simulink model "gm_sampleModel1743_4_sub"  (R2023a)
settings: Solver=VariableStepAuto  StartTime=0.0  StopTime=10.0  RelTol=1e-3
libraries: hdlsllib x3, simulink x2
settings Model: Creator=user1  LastModifiedBy=user1
settings OptimizationCC: BlockReduction=off  ConditionallyExecuteInputs=off
settings DebuggingCC: InheritedTsInSrcMsg=none

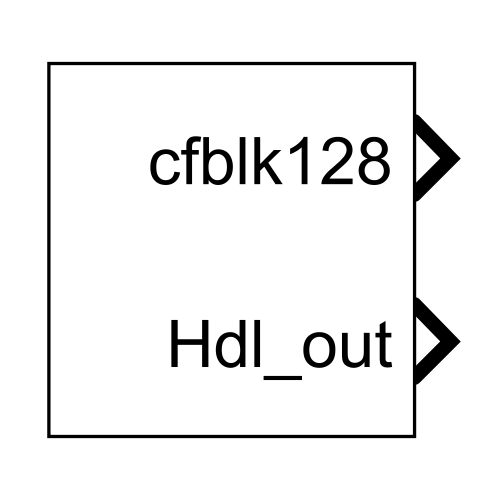
[thumbnail: Simulink's stored preview of the top-level diagram]
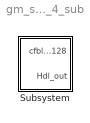
== system gm_sampleModel1743_4_sub ==
  Subsystem : Subsystem

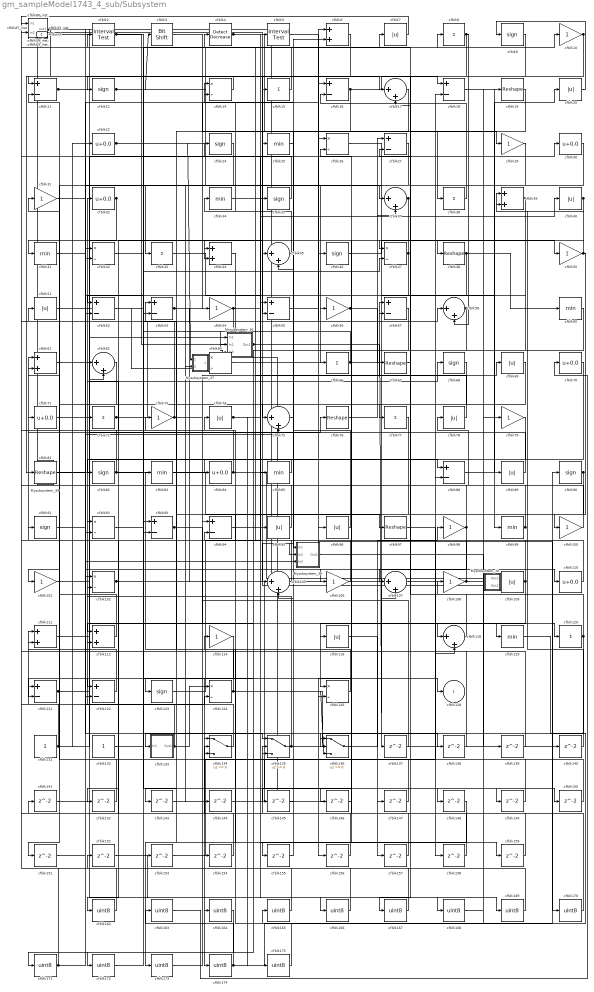
== system gm_sampleModel1743_4_sub/Subsystem ==
  Mysubsystem_16 : Subsystem
  Mysubsystem_19 : Subsystem
  Mysubsystem_36 : Subsystem
  Mysubsystem_37 : Subsystem
  Mysubsystem_39 : Subsystem
  cfblk{10,29,31,50,54,56,73,79,98,100..101,106,108,114} (14 alike) : Gain  OutDataTypeStr=uint8
  cfblk{14,26,42,47,64,92,102,124,126} (9 alike) : Product  Inputs=*/  OutDataTypeStr=uint8  RndMeth=Zero  SaturateOnIntegerOverflow=on
  cfblk104_inst : Subsystem
  cfblk{17,37,45,58,62,75,105,107,118} (9 alike) : Sum  Inputs=|++  OutDataTypeStr=uint8
  cfblk{7,20,40,51,69,74,78,89,95..96,109,116} (12 alike) : Abs  OutDataTypeStr=uint8  SaturateOnIntegerOverflow=off
  cfblk{11,16,18,27,52..53,55,57,88,93..94,121..122} (13 alike) : Sum  Inputs=+-  OutDataTypeStr=uint8
  cfblk{22,30,32,70..71,84,110} (7 alike) : Bias  Bias=0.0  SaturateOnIntegerOverflow=off
  cfblk{6,39,44,61,111..112} (6 alike) : Sum  OutDataTypeStr=uint8
  cfblk117_inst : Subsystem
  cfblk{25,34,41,60,83,85,99,119} (8 alike) : MinMax  OutDataTypeStr=uint8
  cfblk{9,12,24,35,46,68,82,90..91,123} (10 alike) : Signum
  cfblk{8,15,38,43,66,72,77,120} (8 alike) : Sum  Inputs=+  OutDataTypeStr=uint8
  cfblk125_inst : Subsystem
  cfblk131 : Constant  OutDataTypeStr=uint8  SampleTime=-1
  cfblk132 : Constant  OutDataTypeStr=uint8  SampleTime=-1
  cfblk133 : Subsystem
  cfblk134 : Switch  OutDataTypeStr=uint8  SaturateOnIntegerOverflow=off  InputSameDT=off
  cfblk135 : Switch  OutDataTypeStr=uint8  SaturateOnIntegerOverflow=off  InputSameDT=off
  cfblk136 : Switch  OutDataTypeStr=uint8  SaturateOnIntegerOverflow=off  InputSameDT=off
  cfblk{137..159} (23 alike) : Delay  SampleTime=1
  cfblk13_inst : Subsystem
  cfblk{162..175} (14 alike) : DataTypeConversion  OutDataTypeStr=uint8  SaturateOnIntegerOverflow=off  RndMeth=Floor
  cfblk{19,48,67,76,81,97} (6 alike) : Reshape
  cfblk2 : hdlsllib/Logic and Bit Operations/Interval Test  IntervalClosedRight=on  uplimit=0.5  IntervalClosedLeft=on  lowlimit=-0.5  OutDataTypeStr=uint8
  cfblk3 : hdlsllib/Logic and Bit Operations/Bit Shift  mode=Shift Left Logical  N=0
  cfblk33_inst : Subsystem
  cfblk4 : simulink/Logic and Bit Operations/Detect Decrease  vinit=0.0  OutDataTypeStr=uint8
      settings: LibrarySourceBlock=|
      | hdlsllib/Logic and Bit
      | Operations/Detect
      | Decrease
  cfblk5 : hdlsllib/Logic and Bit Operations/Interval Test  IntervalClosedRight=on  uplimit=0.5  IntervalClosedLeft=on  lowlimit=-0.5  OutDataTypeStr=uint8
  cfblk59_inst : Subsystem
  cfblk63_inst : Subsystem
  cfblk80_inst : Subsystem
  cfblk87_inst : Subsystem
  cfblk128 : Outport  OutDataTypeStr=uint8  SampleTime=1  VectorParamsAs1DForOutWhenUnconnected=off
  Hdl_out : Outport  Port=2  OutDataTypeStr=uint8  SampleTime=1
  wires:
  Mysubsystem_16/1(Out1) -> cfblk137/1, Hdl_out/1
  Mysubsystem_19/1(Out1) -> Mysubsystem_39/1(In1)
  Mysubsystem_19/2(Out2) -> cfblk33_inst/2(in2)
  Mysubsystem_36/1(Out1) -> cfblk139/1
  Mysubsystem_37/1(Out1) -> cfblk140/1
  Mysubsystem_39/1(Out1) -> cfblk104_inst/1(in1)
  cfblk10/1 -> cfblk58/2, cfblk55/2
  cfblk100/1 -> cfblk4/1
  cfblk101/1 -> cfblk76/1
  cfblk102/1 -> cfblk168/1, cfblk54/1, cfblk149/1, cfblk148/1
  cfblk104_inst/1(out1) -> cfblk88/1
  cfblk105/1 -> cfblk94/2
  cfblk106/1 -> cfblk34/1
  cfblk107/1 -> cfblk18/2
  cfblk108/1 -> cfblk61/1, cfblk120/1
  cfblk109/1 -> cfblk74/1, cfblk126/1
  cfblk11/1 -> Mysubsystem_16/1(In1), cfblk119/1
  cfblk110/1 -> cfblk87_inst/2(in2)
  cfblk111/1 -> cfblk116/1
  cfblk112/1 -> cfblk51/1
  cfblk114/1 -> cfblk174/1
  cfblk116/1 -> cfblk147/1
  cfblk117_inst/1(out1) -> cfblk164/1
  cfblk118/1 -> cfblk108/1
  cfblk119/1 -> cfblk165/1
  cfblk12/1 -> cfblk3/1, cfblk107/2, cfblk10/1
  cfblk120/1 -> cfblk91/1, cfblk87_inst/1(in1), cfblk133/1(In1)
  cfblk121/1 -> cfblk61/2, cfblk25/1
  cfblk122/1 -> cfblk111/1
  cfblk123/1 -> cfblk55/1
  cfblk124/1 -> cfblk136/3, cfblk157/1, cfblk156/1, cfblk83/1
  cfblk125_inst/1(out1) -> cfblk106/1
  cfblk126/1 -> cfblk53/1
  cfblk13_inst/1(out1) -> cfblk45/1
  cfblk131/1 -> cfblk62/2, cfblk22/1, cfblk111/2
  cfblk132/1 -> cfblk7/1
  cfblk133/1(Out1) -> cfblk125_inst/1(in1), cfblk124/1
  cfblk134/1 -> cfblk32/1
  cfblk135/1 -> cfblk138/1, cfblk102/2
  cfblk136/1 -> cfblk98/1
  cfblk137/1 -> cfblk94/1
  cfblk138/1 -> cfblk13_inst/2(in2)
  cfblk139/1 -> cfblk112/2
  cfblk14/1 -> cfblk11/1
  cfblk140/1 -> cfblk39/1
  cfblk141/1 -> cfblk169/1
  cfblk142/1 -> cfblk102/1
  cfblk143/1 -> cfblk135/2
  cfblk144/1 -> cfblk88/2
  cfblk145/1 -> cfblk6/2
  cfblk146/1 -> cfblk64/1
  cfblk147/1 -> cfblk11/2
  cfblk148/1 -> cfblk173/1
  cfblk149/1 -> cfblk105/2
  cfblk15/1 -> cfblk2/1
  cfblk150/1 -> cfblk134/2
  cfblk151/1 -> cfblk42/1
  cfblk152/1 -> cfblk166/1
  cfblk153/1 -> cfblk118/2
  cfblk154/1 -> cfblk104_inst/2(in2)
  cfblk155/1 -> cfblk45/2
  cfblk156/1 -> cfblk92/1
  cfblk157/1 -> cfblk134/3
  cfblk158/1 -> cfblk26/2
  cfblk159/1 -> cfblk135/3
  cfblk16/1 -> cfblk18/1, cfblk143/1
  cfblk162/1 -> cfblk152/1
  cfblk163/1 -> cfblk70/1
  cfblk164/1 -> cfblk172/1
  cfblk165/1 -> cfblk117_inst/1(in1)
  cfblk166/1 -> cfblk117_inst/2(in2)
  cfblk167/1 -> cfblk63_inst/1(in1)
  cfblk168/1 -> cfblk19/1
  cfblk169/1 -> cfblk63_inst/2(in2)
  cfblk17/1 -> cfblk75/1
  cfblk170/1 -> cfblk141/1
  cfblk171/1 -> cfblk33_inst/1(in1), cfblk124/2
  cfblk172/1 -> cfblk57/1
  cfblk173/1 -> cfblk57/2
  cfblk174/1 -> cfblk90/1, cfblk163/1, cfblk79/1
  cfblk175/1 -> cfblk114/1
  cfblk18/1 -> cfblk89/1
  cfblk19/1 -> cfblk167/1
  cfblk2/1 -> cfblk150/1, cfblk128/1
  cfblk20/1 -> cfblk9/1
  cfblk22/1 -> cfblk96/1, Mysubsystem_37/1(In1)
  cfblk24/1 -> cfblk43/1
  cfblk25/1 -> Mysubsystem_36/1(In1)
  cfblk26/1 -> cfblk99/1
  cfblk27/1 -> cfblk66/1
  cfblk29/1 -> Mysubsystem_37/2(In2)
  cfblk3/1 -> cfblk29/1
  cfblk30/1 -> cfblk151/1
  cfblk31/1 -> cfblk53/2
  cfblk32/1 -> cfblk121/2, cfblk42/2, cfblk41/1
  cfblk33_inst/1(out1) -> cfblk72/1
  cfblk34/1 -> cfblk95/1
  cfblk35/1 -> cfblk13_inst/1(in1)
  cfblk37/1 -> cfblk142/1, cfblk126/2
  cfblk38/1 -> cfblk16/2
  cfblk39/1 -> cfblk52/1, cfblk112/1
  cfblk4/1 -> cfblk146/1, cfblk38/1
  cfblk40/1 -> cfblk39/2, cfblk136/2
  cfblk41/1 -> cfblk15/1
  cfblk42/1 -> cfblk93/1
  cfblk43/1 -> cfblk85/1
  cfblk44/1 -> Mysubsystem_16/2(In2)
  cfblk45/1 -> cfblk14/1
  cfblk46/1 -> cfblk50/1
  cfblk47/1 -> cfblk44/2, cfblk44/1, cfblk56/1
  cfblk48/1 -> cfblk123/1, Mysubsystem_36/2(In2), cfblk60/1
  cfblk5/1 -> cfblk170/1
  cfblk50/1 -> cfblk47/1, cfblk100/1
  cfblk51/1 -> cfblk64/2
  cfblk52/1 -> cfblk8/1
  cfblk53/1 -> cfblk16/1, cfblk144/1
  cfblk54/1 -> cfblk93/2, cfblk26/1, cfblk159/1
  cfblk55/1 -> cfblk46/1
  cfblk56/1 -> cfblk67/1, cfblk145/1
  cfblk57/1 -> cfblk171/1
  cfblk58/1 -> cfblk122/1, cfblk121/1
  cfblk59_inst/1(out1) -> cfblk37/1, cfblk109/1
  cfblk6/1 -> cfblk92/2
  cfblk60/1 -> cfblk82/1
  cfblk61/1 -> cfblk68/1
  cfblk62/1 -> cfblk122/2
  cfblk63_inst/1(out1) -> cfblk52/2, Mysubsystem_36/3(In3)
  cfblk64/1 -> cfblk35/1
  cfblk66/1 -> cfblk37/2, Mysubsystem_16/3(In3)
  cfblk67/1 -> cfblk27/2
  cfblk68/1 -> cfblk101/1
  cfblk69/1 -> cfblk136/1
  cfblk7/1 -> cfblk80_inst/1(in1)
  cfblk70/1 -> cfblk162/1
  cfblk71/1 -> cfblk110/1
  cfblk72/1 -> cfblk6/1, cfblk58/1
  cfblk73/1 -> cfblk69/1, cfblk125_inst/2(in2)
  cfblk74/1 -> cfblk30/1, cfblk175/1
  cfblk75/1 -> cfblk5/1
  cfblk76/1 -> cfblk27/1
  cfblk77/1 -> cfblk105/1
  cfblk78/1 -> cfblk24/1
  cfblk79/1 -> cfblk155/1
  cfblk8/1 -> cfblk48/1, cfblk12/1
  cfblk80_inst/1(out1) -> cfblk81/1
  cfblk81/1 -> cfblk134/1
  cfblk82/1 -> cfblk47/2, cfblk31/1
  cfblk83/1 -> cfblk97/1
  cfblk84/1 -> cfblk80_inst/2(in2), cfblk62/1
  cfblk85/1 -> cfblk84/1
  cfblk87_inst/1(out1) -> cfblk17/1
  cfblk88/1 -> cfblk20/1
  cfblk89/1 -> cfblk71/1
  cfblk9/1 -> cfblk77/1
  cfblk90/1 -> cfblk154/1, cfblk153/1
  cfblk91/1 -> cfblk75/2
  cfblk92/1 -> cfblk135/1
  cfblk93/1 -> cfblk118/1, cfblk73/1
  cfblk94/1 -> cfblk40/1
  cfblk95/1 -> cfblk59_inst/1(in1)
  cfblk96/1 -> cfblk14/2
  cfblk97/1 -> cfblk158/1
  cfblk98/1 -> cfblk17/2, cfblk107/1
  cfblk99/1 -> cfblk78/1, cfblk59_inst/2(in2)

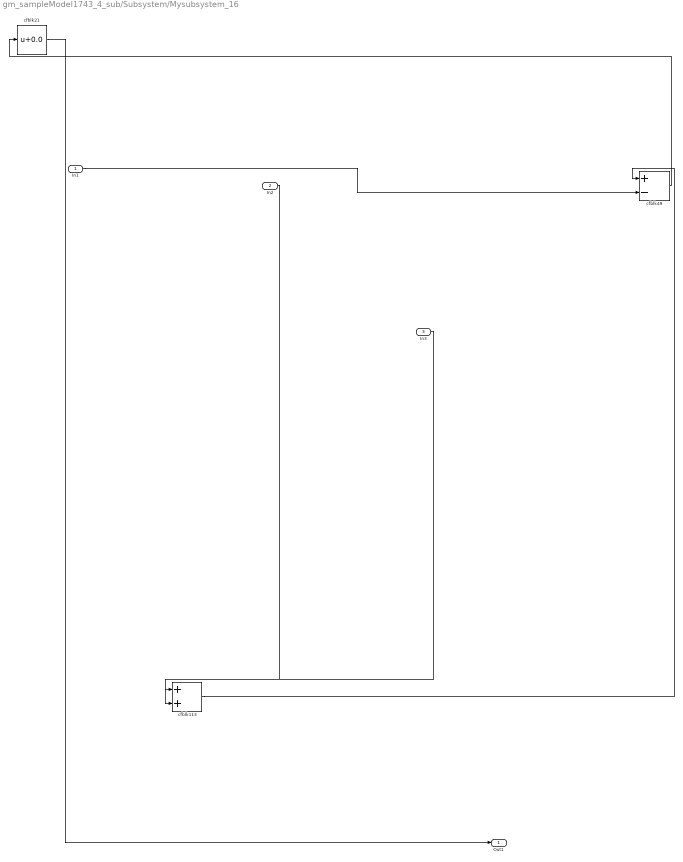
== system gm_sampleModel1743_4_sub/Subsystem/Mysubsystem_16 ==
  In1 : Inport  OutDataTypeStr=uint8  PortDimensions=1  SampleTime=1
  In2 : Inport  Port=2  OutDataTypeStr=uint8  PortDimensions=1  SampleTime=1
  In3 : Inport  Port=3  OutDataTypeStr=uint8  PortDimensions=1  SampleTime=1
  cfblk113 : Sum
  cfblk21 : Bias  Bias=0.0  SaturateOnIntegerOverflow=off
  cfblk49 : Sum  Inputs=+-
  Out1 : Outport  SampleTime=1
  wires:
  In1/1 -> cfblk49/2
  In2/1 -> cfblk113/2
  In3/1 -> cfblk113/1
  cfblk113/1 -> cfblk49/1
  cfblk21/1 -> Out1/1
  cfblk49/1 -> cfblk21/1

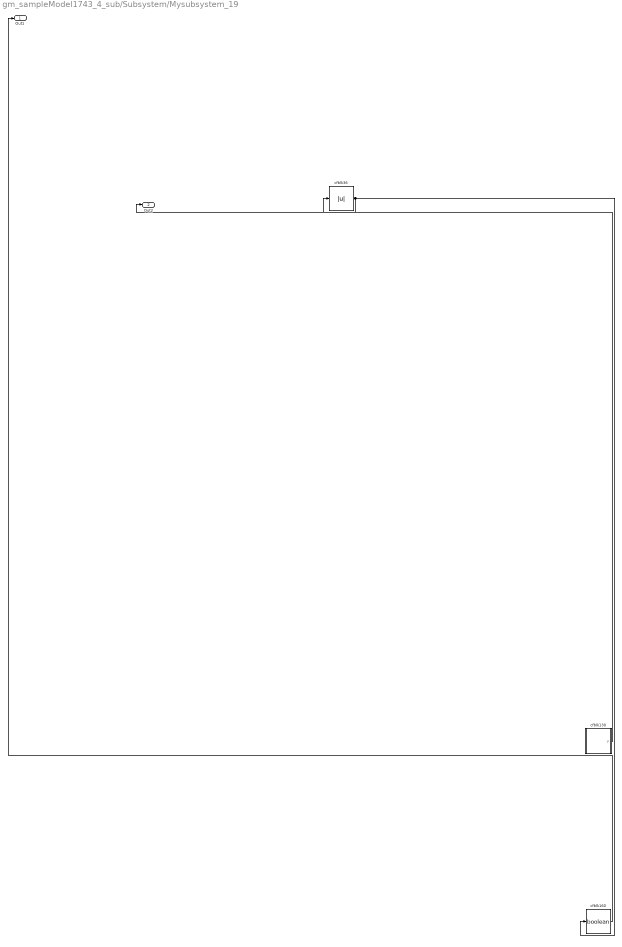
== system gm_sampleModel1743_4_sub/Subsystem/Mysubsystem_19 ==
  cfblk130 : Subsystem  mask(Counter Limited){uplimit=double(7), tsamp=double(-1)}
      mask prompts: uplimit "Simulink:masks:UpperLimit_MP"; tsamp "Simulink:masks:SampleTime_MP"
      mask help: Simulink:masks:CounterLimited_MD
      mask init:
      | nbits = double(8);
      | tsamp = double(-1);
      | uplimit = double(7);
  cfblk160 : DataTypeConversion  OutDataTypeStr=boolean  SaturateOnIntegerOverflow=off  RndMeth=Floor
  cfblk36 : Abs  SaturateOnIntegerOverflow=off
  Out1 : Outport  SampleTime=1
  Out2 : Outport  Port=2  SampleTime=1
  wires:
  cfblk130/1(y) -> cfblk36/1
  cfblk160/1 -> Out1/1
  cfblk36/1 -> cfblk160/1, Out2/1

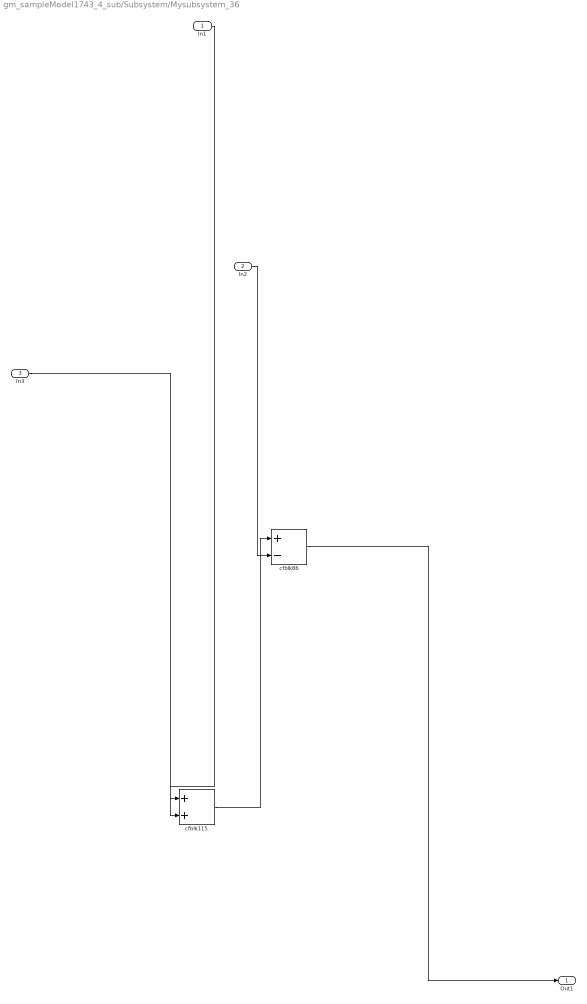
== system gm_sampleModel1743_4_sub/Subsystem/Mysubsystem_36 ==
  In1 : Inport  OutDataTypeStr=uint8  PortDimensions=1  SampleTime=1
  In2 : Inport  Port=2  OutDataTypeStr=uint8  PortDimensions=1  SampleTime=1
  In3 : Inport  Port=3  OutDataTypeStr=uint8  PortDimensions=1  SampleTime=1
  cfblk115 : Sum
  cfblk86 : Sum  Inputs=+-
  Out1 : Outport  SampleTime=1
  wires:
  In1/1 -> cfblk115/2
  In2/1 -> cfblk86/2
  In3/1 -> cfblk115/1
  cfblk115/1 -> cfblk86/1
  cfblk86/1 -> Out1/1

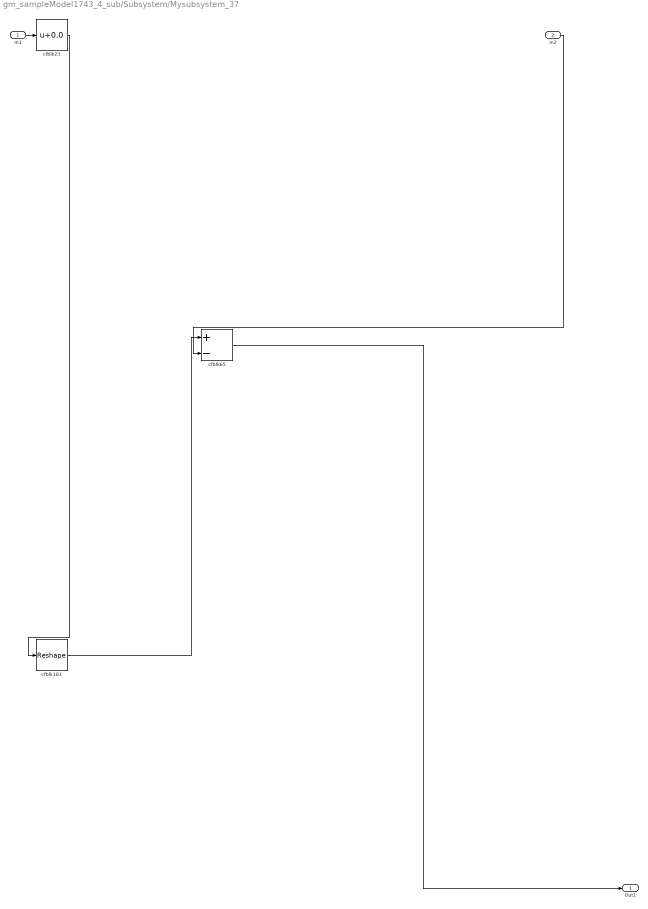
== system gm_sampleModel1743_4_sub/Subsystem/Mysubsystem_37 ==
  In1 : Inport  OutDataTypeStr=uint8  PortDimensions=1  SampleTime=1
  In2 : Inport  Port=2  OutDataTypeStr=uint8  PortDimensions=1  SampleTime=1
  cfblk103 : Reshape
  cfblk23 : Bias  Bias=0.0  SaturateOnIntegerOverflow=off
  cfblk65 : Sum  Inputs=+-
  Out1 : Outport  SampleTime=1
  wires:
  In1/1 -> cfblk23/1
  In2/1 -> cfblk65/2
  cfblk103/1 -> cfblk65/1
  cfblk23/1 -> cfblk103/1
  cfblk65/1 -> Out1/1

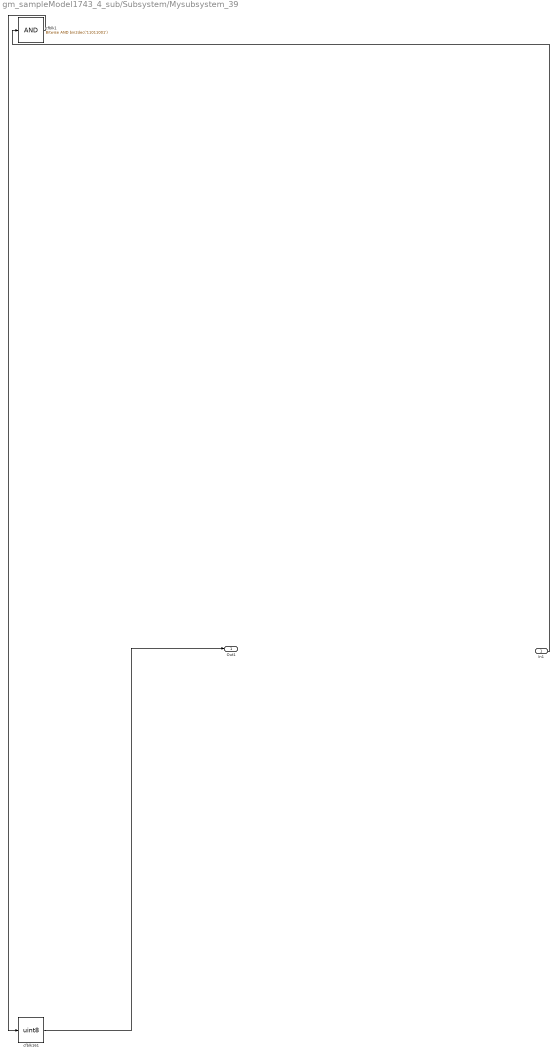
== system gm_sampleModel1743_4_sub/Subsystem/Mysubsystem_39 ==
  In1 : Inport  OutDataTypeStr=boolean  PortDimensions=1  SampleTime=1
  cfblk1 : simulink/Logic and Bit Operations/Bitwise Operator  logicop=AND  UseBitMask=on  BitMask=bin2dec('11011001')  BitMaskRealWorld=Stored Integer
      settings: LibrarySourceBlock=|
      | hdlsllib/Logic and Bit
      | Operations/Bitwise
      | Operator
  cfblk161 : DataTypeConversion  OutDataTypeStr=uint8  SaturateOnIntegerOverflow=off  RndMeth=Floor
  Out1 : Outport  SampleTime=1
  wires:
  In1/1 -> cfblk1/1
  cfblk1/1 -> cfblk161/1
  cfblk161/1 -> Out1/1

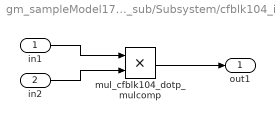
== system gm_sampleModel1743_4_sub/Subsystem/cfblk104_inst ==
  in1 : Inport  OutDataTypeStr=uint8  SampleTime=1
  in2 : Inport  Port=2  OutDataTypeStr=uint8  SampleTime=1
  mul_cfblk104_dotp_mulcomp : Product  Inputs=**  OutDataTypeStr=uint8  SampleTime=1
  out1 : Outport  OutDataTypeStr=uint8  SampleTime=1
  wires:
  in1/1 -> mul_cfblk104_dotp_mulcomp/1
  in2/1 -> mul_cfblk104_dotp_mulcomp/2
  mul_cfblk104_dotp_mulcomp/1 -> out1/1

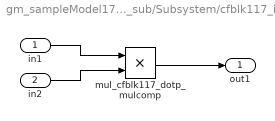
== system gm_sampleModel1743_4_sub/Subsystem/cfblk117_inst ==
  in1 : Inport  OutDataTypeStr=uint8  SampleTime=1
  in2 : Inport  Port=2  OutDataTypeStr=uint8  SampleTime=1
  mul_cfblk117_dotp_mulcomp : Product  Inputs=**  OutDataTypeStr=uint8  SampleTime=1
  out1 : Outport  OutDataTypeStr=uint8  SampleTime=1
  wires:
  in1/1 -> mul_cfblk117_dotp_mulcomp/1
  in2/1 -> mul_cfblk117_dotp_mulcomp/2
  mul_cfblk117_dotp_mulcomp/1 -> out1/1

== system gm_sampleModel1743_4_sub/Subsystem/cfblk125_inst ==
  in1 : Inport  OutDataTypeStr=uint8  SampleTime=1
  in2 : Inport  Port=2  OutDataTypeStr=uint8  SampleTime=1
  mul_cfblk125_dotp_mulcomp : Product  Inputs=**  OutDataTypeStr=uint8  SampleTime=1
  out1 : Outport  OutDataTypeStr=uint8  SampleTime=1
  wires:
  in1/1 -> mul_cfblk125_dotp_mulcomp/1
  in2/1 -> mul_cfblk125_dotp_mulcomp/2
  mul_cfblk125_dotp_mulcomp/1 -> out1/1

== system gm_sampleModel1743_4_sub/Subsystem/cfblk133 ==
  In1 : Inport  OutDataTypeStr=uint8  PortDimensions=1  SampleTime=1
  Out1 : Outport  SampleTime=1
  wires:
  In1/1 -> Out1/1

== system gm_sampleModel1743_4_sub/Subsystem/cfblk13_inst ==
  in1 : Inport  OutDataTypeStr=uint8  SampleTime=1
  in2 : Inport  Port=2  OutDataTypeStr=uint8  SampleTime=1
  mul_cfblk13_dotp_mulcomp : Product  Inputs=**  OutDataTypeStr=uint8  SampleTime=1
  out1 : Outport  OutDataTypeStr=uint8  SampleTime=1
  wires:
  in1/1 -> mul_cfblk13_dotp_mulcomp/1
  in2/1 -> mul_cfblk13_dotp_mulcomp/2
  mul_cfblk13_dotp_mulcomp/1 -> out1/1

== system gm_sampleModel1743_4_sub/Subsystem/cfblk33_inst ==
  in1 : Inport  OutDataTypeStr=uint8  SampleTime=1
  in2 : Inport  Port=2  OutDataTypeStr=uint8  SampleTime=1
  mul_cfblk33_dotp_mulcomp : Product  Inputs=**  OutDataTypeStr=uint8  SampleTime=1
  out1 : Outport  OutDataTypeStr=uint8  SampleTime=1
  wires:
  in1/1 -> mul_cfblk33_dotp_mulcomp/1
  in2/1 -> mul_cfblk33_dotp_mulcomp/2
  mul_cfblk33_dotp_mulcomp/1 -> out1/1

== system gm_sampleModel1743_4_sub/Subsystem/cfblk59_inst ==
  in1 : Inport  OutDataTypeStr=uint8  SampleTime=1
  in2 : Inport  Port=2  OutDataTypeStr=uint8  SampleTime=1
  mul_cfblk59_dotp_mulcomp : Product  Inputs=**  OutDataTypeStr=uint8  SampleTime=1
  out1 : Outport  OutDataTypeStr=uint8  SampleTime=1
  wires:
  in1/1 -> mul_cfblk59_dotp_mulcomp/1
  in2/1 -> mul_cfblk59_dotp_mulcomp/2
  mul_cfblk59_dotp_mulcomp/1 -> out1/1

== system gm_sampleModel1743_4_sub/Subsystem/cfblk63_inst ==
  in1 : Inport  OutDataTypeStr=uint8  SampleTime=1
  in2 : Inport  Port=2  OutDataTypeStr=uint8  SampleTime=1
  mul_cfblk63_dotp_mulcomp : Product  Inputs=**  OutDataTypeStr=uint8  SampleTime=1
  out1 : Outport  OutDataTypeStr=uint8  SampleTime=1
  wires:
  in1/1 -> mul_cfblk63_dotp_mulcomp/1
  in2/1 -> mul_cfblk63_dotp_mulcomp/2
  mul_cfblk63_dotp_mulcomp/1 -> out1/1

== system gm_sampleModel1743_4_sub/Subsystem/cfblk80_inst ==
  in1 : Inport  OutDataTypeStr=uint8  SampleTime=1
  in2 : Inport  Port=2  OutDataTypeStr=uint8  SampleTime=1
  mul_cfblk80_dotp_mulcomp : Product  Inputs=**  OutDataTypeStr=uint8  SampleTime=1
  out1 : Outport  OutDataTypeStr=uint8  SampleTime=1
  wires:
  in1/1 -> mul_cfblk80_dotp_mulcomp/1
  in2/1 -> mul_cfblk80_dotp_mulcomp/2
  mul_cfblk80_dotp_mulcomp/1 -> out1/1

== system gm_sampleModel1743_4_sub/Subsystem/cfblk87_inst ==
  in1 : Inport  OutDataTypeStr=uint8  SampleTime=1
  in2 : Inport  Port=2  OutDataTypeStr=uint8  SampleTime=1
  mul_cfblk87_dotp_mulcomp : Product  Inputs=**  OutDataTypeStr=uint8  SampleTime=1
  out1 : Outport  OutDataTypeStr=uint8  SampleTime=1
  wires:
  in1/1 -> mul_cfblk87_dotp_mulcomp/1
  in2/1 -> mul_cfblk87_dotp_mulcomp/2
  mul_cfblk87_dotp_mulcomp/1 -> out1/1

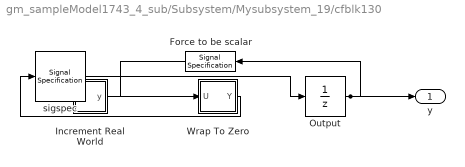
== system gm_sampleModel1743_4_sub/Subsystem/Mysubsystem_19/cfblk130 ==
  Force to be scalar : SignalSpecification  DisableCoverage=on  Dimensions=1
  Increment Real World : Subsystem  mask(Real World Value Increment){}
      mask help: Simulink:masks:RealWorldValueIncrement_MD
      mask Display: disp('V++')
  Output : UnitDelay  InitialCondition=0.0  SampleTime=tsamp  HasFrameUpgradeWarning=on
  Wrap To Zero : Subsystem  mask(Wrap To Zero){Threshold=double(7)}
      mask prompts: Threshold "Simulink:masks:Threshold_MP"
      mask help: Simulink:masks:WrapToZero_MD
  sigspec : SignalSpecification  OutDataTypeStr=uint8  Dimensions=1
  y : Outport  SampleTime=1
  wires:
  Force to be scalar/1 -> Increment Real World/1(u)
  Increment Real World/1(y) -> Wrap To Zero/1(U)
  Output/1 -> Force to be scalar/1, y/1
  Wrap To Zero/1(Y) -> sigspec/1
  sigspec/1 -> Output/1

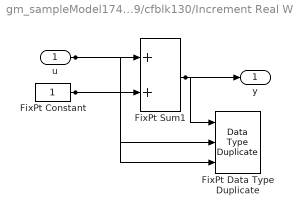
== system gm_sampleModel1743_4_sub/Subsystem/Mysubsystem_19/cfblk130/Increment Real World ==
  u : Inport  OutDataTypeStr=uint8  SampleTime=1
  FixPt Constant : Constant  DisableCoverage=on  OutDataTypeStr=Inherit: Inherit via back propagation  SampleTime=-1
  FixPt Data Type Duplicate : DataTypeDuplicate  DisableCoverage=on  NumInputPorts=3
  FixPt Sum1 : Sum  InputSameDT=on  OutDataTypeStr=Inherit: Inherit via back propagation  LockScale=on
  y : Outport  SampleTime=1
  wires:
  u/1 -> FixPt Sum1/1, FixPt Data Type Duplicate/2
  FixPt Constant/1 -> FixPt Sum1/2, FixPt Data Type Duplicate/3
  FixPt Sum1/1 -> FixPt Data Type Duplicate/1, y/1

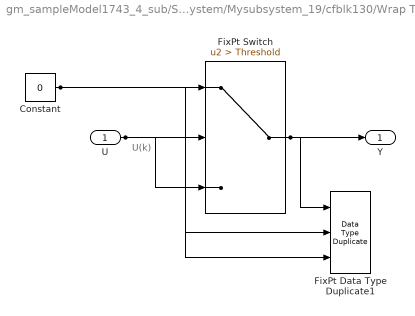
== system gm_sampleModel1743_4_sub/Subsystem/Mysubsystem_19/cfblk130/Wrap To Zero ==
  note: U(k)
  U : Inport  OutDataTypeStr=uint8  SampleTime=1
  Constant : Constant  DisableCoverage=on  Value=0  OutDataTypeStr=Inherit: Inherit via back propagation  SampleTime=-1
  FixPt Data Type Duplicate1 : DataTypeDuplicate  DisableCoverage=on  NumInputPorts=3
  FixPt Switch : Switch  Criteria=u2 > Threshold  Threshold=Threshold  OutDataTypeStr=Inherit: Inherit via back propagation  ZeroCross=off  SaturateOnIntegerOverflow=off  InputSameDT=off
  Y : Outport  SampleTime=1
  wires:
  U/1 -> FixPt Switch/3, FixPt Switch/2, FixPt Data Type Duplicate1/2
  Constant/1 -> FixPt Switch/1, FixPt Data Type Duplicate1/3
  FixPt Switch/1 -> FixPt Data Type Duplicate1/1, Y/1
